simulink model "Step1"  (R2017b)
settings: Solver=FixedStepDiscrete  StartTime=0.0  StopTime=10.0  FixedStep=1.000000  RelTol=1e-3  EnableMultiTasking=on
model workspace (MAT data in the model file):
  already_pp = 0
  input_struct.time = [0; 1; 2; 3; 4; 5; 6; 7; 8; 9; 10; 11; 12; 13; 14; 15; 16; 17; 18; 19; 20; 21; 22; 23; 24; 25; 26; 27; 28; 29; 30; 31; 32; 33; 34; 35; 36; 37; 38; 39; 40; 41; 42; 43; 44; 45; 46; 47; 48; 49; 50; 51; 52; 53; 54; 55; 56; 57; 58; 59; 60; 61; 62; 63; 64; 65; 66; 67; 68; 69; 70; 71; 72; 73; 74; 75; 76; 77; 78; 79; 80; 81; 82; 83; 84; 85; 86; 87; 88; 89; 90; 91; 92; 93; 94; 95; 96; 97; 98; 99]
  input_struct.signals(1).name = 'x'
  input_struct.signals(1).values = [-100  52  2; 97  9  -67; 14  -29  43; -31  40  82; 12  -79  -57; -40  -99  75; -69  20  -58; 33  32  68; 37  16  72; 59  82  5; -30  27  -5; -50  5  78; -31  -48  -87; -34  -90  2; 86  47  24; 51  -67  47; -43  -44  -54; 21  -48  -96; 53  9  -73; 70  8  54; 81  58  94; 19  74  -23; -87  58  99; -57  94  -35; 74  -64  -73; -17  87  -23; 32  -91  13; 57  -52  27; -51  -99  8; 11  34  -37; -54  81  -68; -99  15  -70; 54  -69  -73; -96  0  42; -21  14  -7; -50  -63  -78; -59  -35  40; 33  43  -64; 83  11  61; -99  -72  3; 50  -24  10; 60  -21  -59; 82  15  57; 95  -97  5; -76  16  14; 4  87  -16; 65  -79  44; 28  47  -86; 91  95  19; 90  22  73; 94  44  -10; -87  -40  31; -13  -8  -40; -36  -91  22; -74  -23  -44; -73  -28  60; 61  -43  60; 5  64  91; 89  -10  -11; 98  62  -9; -18  58  20; -26  -44  69; -55  -87  -94; -11  -89  -63; -47  28  89; -8  -15  90; -13  82  -9; -48  -17  62; -74  -70  86; -16  8  35; 1  88  -26; -35  32  -19; 37  -21  -12; -11  -48  36; -13  70  -7; 59  89  91; 63  -25  -29; 51  -87  -32; 58  -64  80; 0  15  9; 11  -63  50; 26  -42  -75; -81  -8  -9; -51  -31  -85; 23  -37  33; -39  -8  41; 54  -53  84; -47  -95  32; -93  32  38; -41  -69  71; 11  61  -6; 94  -18  -8; 38  -35  62; 44  49  65; 12  50  -62; 7  -66  -95; 76  -77  -89; -21  -66  -72; -8  26  -66; -59  69  25]
  input_struct.signals(1).dimensions = 3
  input_struct.signals(2).name = 'x1'
  input_struct.signals(2).values = [-94.0969584552 -5.53354695024 35.6885540734 -77.0422061669 -52.7872152007 -42.1838795698 -65.4487411404 -35.2587754567 60.2220197984 -40.0732601566 55.1251446296 10.5541661137 ... (300 elements, 100x3)]
  input_struct.signals(2).dimensions = 3
  input_struct.signals(3).name = 'x2'
  input_struct.signals(3).values = [0  1  1; 0  0  0; 1  1  0; 1  1  1; 0  0  1; 1  1  0; 1  1  1; 1  0  0; 0  1  1; 0  0  1; 0  1  0; 0  0  0; 0  0  1; 1  1  1; 0  1  0; 0  1  0; 1  1  0; 1  0  1; 0  1  1; 1  0  1; 1  0  0; 1  0  0; 0  1  1; 0  1  0; 0  1  0; 0  1  0; 0  1  1; 0  0  0; 1  0  0; 0  0  1; 0  1  1; 1  0  1; 0  1  0; 0  0  1; 1  0  1; 1  0  1; 0  0  0; 1  1  1; 0  1  0; 1  1  1; 1  1  1; 0  1  0; 0  1  0; 0  0  0; 0  0  0; 0  0  0; 1  0  1; 1  0  0; 0  0  1; 1  0  1; 0  1  1; 1  0  1; 1  0  0; 1  0  1; 0  0  1; 1  1  1; 0  0  1; 0  0  1; 0  1  1; 1  0  0; 0  0  0; 0  0  1; 0  1  0; 1  0  1; 1  0  0; 1  1  1; 1  0  0; 0  1  1; 0  1  0; 1  0  1; 0  1  0; 1  1  0; 1  1  1; 0  1  0; 0  1  0; 0  0  1; 1  0  0; 1  1  1; 0  1  1; 1  1  1; 0  0  1; 1  1  0; 1  0  0; 0  1  0; 0  1  1; 1  1  0; 1  0  0; 1  1  0; 0  1  0; 0  0  0; 1  0  0; 1  0  0; 0  1  1; 1  1  1; 1  0  0; 0  1  0; 0  0  0; 0  0  0; 0  0  0; 0  0  1]
  input_struct.signals(3).dimensions = 3
settings Model: Creator=Teme  LastModifiedBy=hbourbou
settings DataIOCC: LimitDataPoints=on  SaveFormat=Structure
settings OptimizationCC: LifeSpan=inf
settings DebuggingCC: AlgebraicLoopMsg=error  ArtificialAlgebraicLoopMsg=error  SFUnexpectedBacktrackingDiag=warning  SFNoUnconditionalDefaultTransitionDiag=warning  SFExecutionAtInitializationDiag=none
settings HardwareCC: ProdBitPerPointer=32  ProdBitPerSizeT=32  ProdBitPerPtrDiffT=32  ProdLargestAtomicFloat=None  ProdIntDivRoundTo=Undefined  ProdEndianess=Unspecified  ProdWordSize=32  ProdHWDeviceType=32-bit Generic
settings ModelReferenceCC: PropagateSignalLabelsOutOfModel=off
settings RTWCC: Toolchain=Clang v3.1 | gmake (64-bit Mac)
settings CodeAppCC: StateflowObjectComments=on
settings GRTTargetCC: TargetLangStandard=C89/C90 (ANSI)  GeneratePreprocessorConditionals=Disable all
settings ConfigComp: CovMetricSettings=dw  CovHtmlReporting=on  CovSaveCumulativeToWorkspaceVar=on  CovSaveSingleToWorkspaceVar=on  CovExternalEMLEnable=off

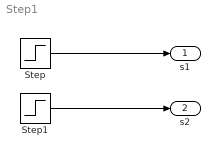
== system Step1 ==
  Step : Step  Time=5  Before=1  After=0  SampleTime=1
  Step1 : Step  Time=10  After=180  SampleTime=1
  s1 : Outport
  s2 : Outport  Port=2
  wires:
  Step/1 -> s1/1
  Step1/1 -> s2/1
